simulink model "step_control_test"  (R2023a)
settings: Solver=VariableStepAuto  StartTime=0.0  StopTime=10.0  RelTol=1e-3
settings Model: Creator=acer  LastModifiedBy=acer

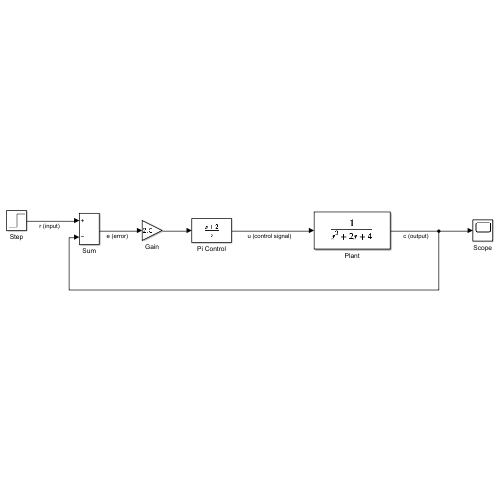
[thumbnail: Simulink's stored preview of the top-level diagram]
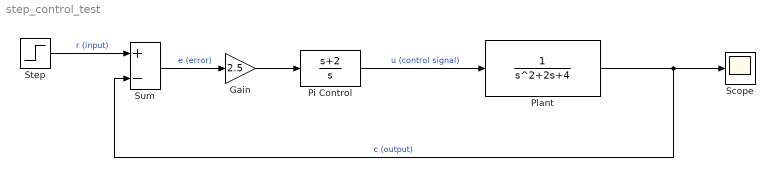
== system step_control_test ==
  Gain : Gain  Gain=2.5
  Pi Control : TransferFcn  Numerator=[1 2]  Denominator=[1 0]
  Plant : TransferFcn  Denominator=[1 2 4]
  Scope : Scope
  Step : Step  SampleTime=0
  Sum : Sum  Inputs=+-
  wires:
  Step/1 -> Sum/1  "r (input)"
  Sum/1 -> Gain/1  "e (error)"
  Gain/1 -> Pi Control/1
  Pi Control/1 -> Plant/1  "u (control signal)"
  Plant/1 -> Sum/2, Scope/1  "c (output)"
